simulink model "HANcoder_E407_TTA_Controller_v4_7"  (R2018b)
settings: Solver=FixedStepDiscrete  StartTime=0.0  StopTime=1  FixedStep=0.01  RelTol=1e-3
PreLoadFcn:
  | librarySetup
  | eval([bdroot,'_startup']) %Calling [modelName]_startup.m
values from neighbouring files (symbols this model uses):
  Backup_Board = 0    [HANcoder_E407_TTA_Controller_v3_5_startup.m]    (also in HANcoder_E407_TTA_Controller_v4_6_startup.m; HANcoder_E407_TTA_Controller_v4_7_startup.m; HANcoder_E407_TTA_Controller_v4_startup.m)
  basic_cycle_duration_bc0 = TM_Reset_Board   + COMP_duration    (= 212)    [HANcoder_E407_TTA_Controller_v3_5_startup.m]    (also in HANcoder_E407_TTA_Controller_v4_6_startup.m; HANcoder_E407_TTA_Controller_v4_7_startup.m; HANcoder_E407_TTA_Controller_v4_startup.m)
  basic_cycle_duration_bc1 = TM_Reset_Var_bc1 + COMP_duration    (= 288)    [HANcoder_E407_TTA_Controller_v3_5_startup.m]    (also in HANcoder_E407_TTA_Controller_v4_6_startup.m = 332; HANcoder_E407_TTA_Controller_v4_7_startup.m = 372; HANcoder_E407_TTA_Controller_v4_startup.m = 332)
  comm_delay_estimation1 = round(comm_delay_measured1*hardware_granularity/frequency_IRQ)    [HANcoder_E407_TTA_Controller_v3_5_startup.m]    (also in HANcoder_E407_TTA_Controller_v4_6_startup.m; HANcoder_E407_TTA_Controller_v4_7_startup.m; HANcoder_E407_TTA_Controller_v4_startup.m)
  comm_delay_estimation2 = round(comm_delay_measured2*hardware_granularity/frequency_IRQ)    [HANcoder_E407_TTA_Controller_v3_5_startup.m]    (also in HANcoder_E407_TTA_Controller_v4_6_startup.m; HANcoder_E407_TTA_Controller_v4_7_startup.m; HANcoder_E407_TTA_Controller_v4_startup.m)
  COMM_Period = 40    [HANcoder_E407_TTA_Controller_v3_5_startup.m]    (also in HANcoder_E407_TTA_Controller_v4_6_startup.m; HANcoder_E407_TTA_Controller_v4_7_startup.m; HANcoder_E407_TTA_Controller_v4_startup.m)
  COMM_Phase1 = Simulink.Parameter    [HANcoder_E407_TTA_Controller_v3_5_startup.m]    (also in HANcoder_E407_TTA_Controller_v4_6_startup.m; HANcoder_E407_TTA_Controller_v4_7_startup.m; HANcoder_E407_TTA_Controller_v4_startup.m)
  COMM_Phase2 = Simulink.Parameter    [HANcoder_E407_TTA_Controller_v3_5_startup.m]    (also in HANcoder_E407_TTA_Controller_v4_6_startup.m; HANcoder_E407_TTA_Controller_v4_7_startup.m; HANcoder_E407_TTA_Controller_v4_startup.m)
  COMM_Phase_init1 = Simulink.Parameter    [HANcoder_E407_TTA_Controller_v3_5_startup.m]    (also in HANcoder_E407_TTA_Controller_v4_6_startup.m; HANcoder_E407_TTA_Controller_v4_7_startup.m; HANcoder_E407_TTA_Controller_v4_startup.m)
  COMM_Phase_init2 = Simulink.Parameter    [HANcoder_E407_TTA_Controller_v3_5_startup.m]    (also in HANcoder_E407_TTA_Controller_v4_6_startup.m; HANcoder_E407_TTA_Controller_v4_7_startup.m; HANcoder_E407_TTA_Controller_v4_startup.m)
  COMP_duration = 4    [HANcoder_E407_TTA_Controller_v3_5_startup.m]    (also in HANcoder_E407_TTA_Controller_v4_6_startup.m; HANcoder_E407_TTA_Controller_v4_7_startup.m; HANcoder_E407_TTA_Controller_v4_startup.m)
  Controller1_Board = 1    [HANcoder_E407_TTA_Controller_v3_5_startup.m]    (also in HANcoder_E407_TTA_Controller_v4_6_startup.m; HANcoder_E407_TTA_Controller_v4_7_startup.m; HANcoder_E407_TTA_Controller_v4_startup.m)
  Controller2_Board = 2    [HANcoder_E407_TTA_Controller_v3_5_startup.m]    (also in HANcoder_E407_TTA_Controller_v4_6_startup.m; HANcoder_E407_TTA_Controller_v4_7_startup.m; HANcoder_E407_TTA_Controller_v4_startup.m)
  Controller3_Board = 3    [HANcoder_E407_TTA_Controller_v3_5_startup.m]    (also in HANcoder_E407_TTA_Controller_v4_6_startup.m; HANcoder_E407_TTA_Controller_v4_7_startup.m; HANcoder_E407_TTA_Controller_v4_startup.m)
  delta_a_set = Simulink.Parameter    [HANcoder_E407_TTA_Controller_v3_5_startup.m]    (also in HANcoder_E407_TTA_Controller_v4_6_startup.m; HANcoder_E407_TTA_Controller_v4_7_startup.m; HANcoder_E407_TTA_Controller_v4_startup.m)
  delta_f_set = Simulink.Parameter    [HANcoder_E407_TTA_Controller_v3_5_startup.m]    (also in HANcoder_E407_TTA_Controller_v4_6_startup.m; HANcoder_E407_TTA_Controller_v4_7_startup.m; HANcoder_E407_TTA_Controller_v4_startup.m)
  delta_max = 1    [HANcoder_E407_TTA_Controller_v3_5_startup.m]    (also in HANcoder_E407_TTA_Controller_v4_6_startup.m; HANcoder_E407_TTA_Controller_v4_7_startup.m; HANcoder_E407_TTA_Controller_v4_startup.m)
  delta_min = -1    [HANcoder_E407_TTA_Controller_v3_5_startup.m]    (also in HANcoder_E407_TTA_Controller_v4_6_startup.m; HANcoder_E407_TTA_Controller_v4_7_startup.m; HANcoder_E407_TTA_Controller_v4_startup.m)
  delta_precision = 6    [HANcoder_E407_TTA_Controller_v3_5_startup.m]    (also in HANcoder_E407_TTA_Controller_v4_6_startup.m; HANcoder_E407_TTA_Controller_v4_7_startup.m; HANcoder_E407_TTA_Controller_v4_startup.m)
  e_width = 0.1    [HANcoder_E407_TTA_Controller_v3_5_startup.m]    (also in HANcoder_E407_TTA_Controller_v4_6_startup.m; HANcoder_E407_TTA_Controller_v4_7_startup.m; HANcoder_E407_TTA_Controller_v4_startup.m)
  frequency_IRQ = 100    [HANcoder_E407_2xCAN_TEST_startup.m]    (also in HANcoder_E407_TTA_Controller_v3_5_startup.m; HANcoder_E407_TTA_Controller_v4_6_startup.m; HANcoder_E407_TTA_Controller_v4_7_startup.m; HANcoder_E407_TTA_Controller_v4_startup.m)
  HANtuneOverride = Simulink.Parameter    [HANcoder_E407_2xCAN_TEST_startup.m]    (also in HANcoder_E407_TTA_Controller_v3_5_startup.m; HANcoder_E407_TTA_Controller_v4_6_startup.m; HANcoder_E407_TTA_Controller_v4_7_startup.m; HANcoder_E407_TTA_Controller_v4_startup.m)
  hardware_granularity = 1000000    [HANcoder_E407_2xCAN_TEST_startup.m]    (also in HANcoder_E407_TTA_Controller_v3_5_startup.m; HANcoder_E407_TTA_Controller_v4_6_startup.m; HANcoder_E407_TTA_Controller_v4_7_startup.m; HANcoder_E407_TTA_Controller_v4_startup.m)
  I_a = 2.25    [HANcoder_E407_TTA_Controller_v3_5_startup.m]    (also in HANcoder_E407_TTA_Controller_v4_6_startup.m; HANcoder_E407_TTA_Controller_v4_7_startup.m; HANcoder_E407_TTA_Controller_v4_startup.m)
  I_f = 2.25    [HANcoder_E407_TTA_Controller_v3_5_startup.m]    (also in HANcoder_E407_TTA_Controller_v4_6_startup.m; HANcoder_E407_TTA_Controller_v4_7_startup.m; HANcoder_E407_TTA_Controller_v4_startup.m)
  idle_time_init = basic_cycle_duration_bc0 + basic_cycle_duration_bc1    (= 500)    [HANcoder_E407_TTA_Controller_v3_5_startup.m]    (also in HANcoder_E407_TTA_Controller_v4_6_startup.m = 544; HANcoder_E407_TTA_Controller_v4_7_startup.m = 584; HANcoder_E407_TTA_Controller_v4_startup.m = 544)
  Input_Gen_Board = 4    [HANcoder_E407_TTA_Controller_v3_5_startup.m]    (also in HANcoder_E407_TTA_Controller_v4_6_startup.m; HANcoder_E407_TTA_Controller_v4_7_startup.m; HANcoder_E407_TTA_Controller_v4_startup.m)
  LA_Clock_Gr = 1    [HANcoder_E407_TTA_Controller_v3_5_startup.m]    (also in HANcoder_E407_TTA_Controller_v4_6_startup.m; HANcoder_E407_TTA_Controller_v4_7_startup.m; HANcoder_E407_TTA_Controller_v4_startup.m)
  LA_COMM_dly = 1    [HANcoder_E407_TTA_Controller_v3_5_startup.m]    (also in HANcoder_E407_TTA_Controller_v4_6_startup.m; HANcoder_E407_TTA_Controller_v4_7_startup.m; HANcoder_E407_TTA_Controller_v4_startup.m)
  LA_COMM_Err = 1    [HANcoder_E407_TTA_Controller_v3_5_startup.m]    (also in HANcoder_E407_TTA_Controller_v4_6_startup.m; HANcoder_E407_TTA_Controller_v4_7_startup.m; HANcoder_E407_TTA_Controller_v4_startup.m)
  LA_E_Desync = 1    [HANcoder_E407_TTA_Controller_v3_5_startup.m]    (also in HANcoder_E407_TTA_Controller_v4_6_startup.m; HANcoder_E407_TTA_Controller_v4_7_startup.m; HANcoder_E407_TTA_Controller_v4_startup.m)
  LA_MEX_Flag = 1    [HANcoder_E407_TTA_Controller_v3_5_startup.m]    (also in HANcoder_E407_TTA_Controller_v4_6_startup.m; HANcoder_E407_TTA_Controller_v4_7_startup.m; HANcoder_E407_TTA_Controller_v4_startup.m)
  LA_Task_Act = 1    [HANcoder_E407_TTA_Controller_v3_5_startup.m]    (also in HANcoder_E407_TTA_Controller_v4_6_startup.m; HANcoder_E407_TTA_Controller_v4_7_startup.m; HANcoder_E407_TTA_Controller_v4_startup.m)
  m_v = 100.0    (= 100)    [HANcoder_E407_TTA_Controller_v3_5_startup.m]    (also in HANcoder_E407_TTA_Controller_v4_6_startup.m; HANcoder_E407_TTA_Controller_v4_7_startup.m; HANcoder_E407_TTA_Controller_v4_startup.m)
  Master_Role = 1    [HANcoder_E407_TTA_Controller_v3_5_startup.m]    (also in HANcoder_E407_TTA_Controller_v4_6_startup.m; HANcoder_E407_TTA_Controller_v4_7_startup.m; HANcoder_E407_TTA_Controller_v4_startup.m)
  matrix_cycle_duration = basic_cycle_duration_bc0 + basic_cycle_duration_bc1    (= 500)    [HANcoder_E407_TTA_Controller_v3_5_startup.m]    (also in HANcoder_E407_TTA_Controller_v4_6_startup.m = 544; HANcoder_E407_TTA_Controller_v4_7_startup.m = 584; HANcoder_E407_TTA_Controller_v4_startup.m = 544)
  matrix_rows = 2    [HANcoder_E407_TTA_Controller_v3_5_startup.m]    (also in HANcoder_E407_TTA_Controller_v4_6_startup.m; HANcoder_E407_TTA_Controller_v4_7_startup.m; HANcoder_E407_TTA_Controller_v4_startup.m)
  max_desync = 15    [HANcoder_E407_TTA_Controller_v3_5_startup.m]    (also in HANcoder_E407_TTA_Controller_v4_6_startup.m; HANcoder_E407_TTA_Controller_v4_7_startup.m = 30; HANcoder_E407_TTA_Controller_v4_startup.m)
  max_num_msgs_CAN1 = 2^Tx_bit_number-1    (= 7)    [HANcoder_E407_TTA_Controller_v3_5_startup.m]    (also in HANcoder_E407_TTA_Controller_v4_6_startup.m = 15; HANcoder_E407_TTA_Controller_v4_7_startup.m = 15; HANcoder_E407_TTA_Controller_v4_startup.m)
  max_num_msgs_CAN2 = max_num_msgs_CAN1    (= 7)    [HANcoder_E407_TTA_Controller_v3_5_startup.m]    (also in HANcoder_E407_TTA_Controller_v4_6_startup.m = 15; HANcoder_E407_TTA_Controller_v4_7_startup.m = 15; HANcoder_E407_TTA_Controller_v4_startup.m)
  min_desync = (-1)*max_desync    (= -15)    [HANcoder_E407_TTA_Controller_v3_5_startup.m]    (also in HANcoder_E407_TTA_Controller_v4_6_startup.m; HANcoder_E407_TTA_Controller_v4_7_startup.m = -30; HANcoder_E407_TTA_Controller_v4_startup.m)
  OutControl1_ID = 23    [HANcoder_E407_TTA_Controller_v3_5_startup.m]    (also in HANcoder_E407_TTA_Controller_v4_6_startup.m; HANcoder_E407_TTA_Controller_v4_7_startup.m; HANcoder_E407_TTA_Controller_v4_startup.m)
  OutControl2_ID = 24    [HANcoder_E407_TTA_Controller_v3_5_startup.m]    (also in HANcoder_E407_TTA_Controller_v4_6_startup.m; HANcoder_E407_TTA_Controller_v4_7_startup.m; HANcoder_E407_TTA_Controller_v4_startup.m)
  OutEmulator_ID = 25    [HANcoder_E407_TTA_Controller_v3_5_startup.m]    (also in HANcoder_E407_TTA_Controller_v4_6_startup.m = 26; HANcoder_E407_TTA_Controller_v4_7_startup.m = 26; HANcoder_E407_TTA_Controller_v4_startup.m)
  OutMaster_ID = 25    [HANcoder_E407_TTA_Controller_v4_6_startup.m]    (also in HANcoder_E407_TTA_Controller_v4_7_startup.m; HANcoder_E407_TTA_Controller_v4_startup.m = 26)
  R_al = 0.10    (= 0.1)    [HANcoder_E407_TTA_Controller_v3_5_startup.m]    (also in HANcoder_E407_TTA_Controller_v4_6_startup.m; HANcoder_E407_TTA_Controller_v4_7_startup.m; HANcoder_E407_TTA_Controller_v4_startup.m)
  R_ar = 0.10    (= 0.1)    [HANcoder_E407_TTA_Controller_v3_5_startup.m]    (also in HANcoder_E407_TTA_Controller_v4_6_startup.m; HANcoder_E407_TTA_Controller_v4_7_startup.m; HANcoder_E407_TTA_Controller_v4_startup.m)
  R_fl = 0.10    (= 0.1)    [HANcoder_E407_TTA_Controller_v3_5_startup.m]    (also in HANcoder_E407_TTA_Controller_v4_6_startup.m; HANcoder_E407_TTA_Controller_v4_7_startup.m; HANcoder_E407_TTA_Controller_v4_startup.m)
  R_fr = 0.10    (= 0.1)    [HANcoder_E407_TTA_Controller_v3_5_startup.m]    (also in HANcoder_E407_TTA_Controller_v4_6_startup.m; HANcoder_E407_TTA_Controller_v4_7_startup.m; HANcoder_E407_TTA_Controller_v4_startup.m)
  script_run = Simulink.Parameter    [HANcoder_E407_TTA_Controller_v3_5_startup.m]    (also in HANcoder_E407_TTA_Controller_v4_6_startup.m; HANcoder_E407_TTA_Controller_v4_7_startup.m; HANcoder_E407_TTA_Controller_v4_startup.m)
  SensorValues_ID = 22    [HANcoder_E407_TTA_Controller_v3_5_startup.m]    (also in HANcoder_E407_TTA_Controller_v4_6_startup.m; HANcoder_E407_TTA_Controller_v4_7_startup.m; HANcoder_E407_TTA_Controller_v4_startup.m)
  SetValues_ID = 21    [HANcoder_E407_TTA_Controller_v3_5_startup.m]    (also in HANcoder_E407_TTA_Controller_v4_6_startup.m; HANcoder_E407_TTA_Controller_v4_7_startup.m; HANcoder_E407_TTA_Controller_v4_startup.m)
  Slave_Role = 2    [HANcoder_E407_TTA_Controller_v3_5_startup.m]    (also in HANcoder_E407_TTA_Controller_v4_6_startup.m; HANcoder_E407_TTA_Controller_v4_7_startup.m; HANcoder_E407_TTA_Controller_v4_startup.m)
  speed_k_d = Simulink.Parameter    [HANcoder_E407_TTA_Controller_v3_5_startup.m]    (also in HANcoder_E407_TTA_Controller_v4_6_startup.m; HANcoder_E407_TTA_Controller_v4_7_startup.m; HANcoder_E407_TTA_Controller_v4_startup.m)
  speed_k_i = Simulink.Parameter    [HANcoder_E407_TTA_Controller_v3_5_startup.m]    (also in HANcoder_E407_TTA_Controller_v4_6_startup.m; HANcoder_E407_TTA_Controller_v4_7_startup.m; HANcoder_E407_TTA_Controller_v4_startup.m)
  speed_k_p = Simulink.Parameter    [HANcoder_E407_TTA_Controller_v3_5_startup.m]    (also in HANcoder_E407_TTA_Controller_v4_6_startup.m; HANcoder_E407_TTA_Controller_v4_7_startup.m; HANcoder_E407_TTA_Controller_v4_startup.m)
  speed_max = 10    [HANcoder_E407_TTA_Controller_v3_5_startup.m]    (also in HANcoder_E407_TTA_Controller_v4_6_startup.m; HANcoder_E407_TTA_Controller_v4_7_startup.m; HANcoder_E407_TTA_Controller_v4_startup.m)
  speed_min = -10    [HANcoder_E407_TTA_Controller_v3_5_startup.m]    (also in HANcoder_E407_TTA_Controller_v4_6_startup.m; HANcoder_E407_TTA_Controller_v4_7_startup.m; HANcoder_E407_TTA_Controller_v4_startup.m)
  speed_precision = 3    [HANcoder_E407_TTA_Controller_v3_5_startup.m]    (also in HANcoder_E407_TTA_Controller_v4_6_startup.m; HANcoder_E407_TTA_Controller_v4_7_startup.m; HANcoder_E407_TTA_Controller_v4_startup.m)
  Sync_ID = 1    [HANcoder_E407_TTA_Controller_v3_5_startup.m]    (also in HANcoder_E407_TTA_Controller_v4_6_startup.m; HANcoder_E407_TTA_Controller_v4_7_startup.m; HANcoder_E407_TTA_Controller_v4_startup.m)
  tau_max = 5    [HANcoder_E407_TTA_Controller_v3_5_startup.m]    (also in HANcoder_E407_TTA_Controller_v4_6_startup.m; HANcoder_E407_TTA_Controller_v4_7_startup.m; HANcoder_E407_TTA_Controller_v4_startup.m)
  tau_min = -5    [HANcoder_E407_TTA_Controller_v3_5_startup.m]    (also in HANcoder_E407_TTA_Controller_v4_6_startup.m; HANcoder_E407_TTA_Controller_v4_7_startup.m; HANcoder_E407_TTA_Controller_v4_startup.m)
  tau_range = abs(tau_max) + abs(tau_min)    [HANcoder_E407_TTA_Controller_v3_5_startup.m]    (also in HANcoder_E407_TTA_Controller_v4_6_startup.m; HANcoder_E407_TTA_Controller_v4_7_startup.m; HANcoder_E407_TTA_Controller_v4_startup.m)
  theta_max = (speed_max/R_fr)*matrix_cycle_duration*frequency_IRQ/hardware_granularity    (= 5)    [HANcoder_E407_TTA_Controller_v3_5_startup.m]    (also in HANcoder_E407_TTA_Controller_v4_6_startup.m = 5.44; HANcoder_E407_TTA_Controller_v4_7_startup.m = 5.84; HANcoder_E407_TTA_Controller_v4_startup.m = 5.44)
  theta_min = (-1)*theta_max    (= -5)    [HANcoder_E407_TTA_Controller_v3_5_startup.m]    (also in HANcoder_E407_TTA_Controller_v4_6_startup.m = -5.44; HANcoder_E407_TTA_Controller_v4_7_startup.m = -5.84; HANcoder_E407_TTA_Controller_v4_startup.m = -5.44)
  theta_precision = 7-(fix(log2(theta_max))+1)    [HANcoder_E407_TTA_Controller_v3_5_startup.m]    (also in HANcoder_E407_TTA_Controller_v4_6_startup.m; HANcoder_E407_TTA_Controller_v4_7_startup.m; HANcoder_E407_TTA_Controller_v4_startup.m)
  Tl_a = 0.6    [HANcoder_E407_TTA_Controller_v3_5_startup.m]    (also in HANcoder_E407_TTA_Controller_v4_6_startup.m; HANcoder_E407_TTA_Controller_v4_7_startup.m; HANcoder_E407_TTA_Controller_v4_startup.m)
  Tl_f = 0.6    [HANcoder_E407_TTA_Controller_v3_5_startup.m]    (also in HANcoder_E407_TTA_Controller_v4_6_startup.m; HANcoder_E407_TTA_Controller_v4_7_startup.m; HANcoder_E407_TTA_Controller_v4_startup.m)
  TM_Check_Output_Control1 = TM_COMM_Output_Control1 + COMM_duration    (= 188)    [HANcoder_E407_TTA_Controller_v3_5_startup.m]    (also in HANcoder_E407_TTA_Controller_v4_6_startup.m; HANcoder_E407_TTA_Controller_v4_7_startup.m; HANcoder_E407_TTA_Controller_v4_startup.m)
  TM_Check_Output_Control2 = TM_COMM_Output_Control2 + COMM_duration    (= 232)    [HANcoder_E407_TTA_Controller_v3_5_startup.m]    (also in HANcoder_E407_TTA_Controller_v4_6_startup.m; HANcoder_E407_TTA_Controller_v4_7_startup.m; HANcoder_E407_TTA_Controller_v4_startup.m)
  TM_Check_Output_Emulator = TM_COMM_Output_Emulator + COMM_duration    (= 280)    [HANcoder_E407_TTA_Controller_v3_5_startup.m]    (also in HANcoder_E407_TTA_Controller_v4_6_startup.m = 320; HANcoder_E407_TTA_Controller_v4_7_startup.m = 360; HANcoder_E407_TTA_Controller_v4_startup.m = 320)
  TM_Check_Output_Emulator_2 = TM_Check_Output_Emulator + 2    (= 282)    [HANcoder_E407_TTA_Controller_v3_5_startup.m]    (also in HANcoder_E407_TTA_Controller_v4_6_startup.m = 322; HANcoder_E407_TTA_Controller_v4_7_startup.m = 362; HANcoder_E407_TTA_Controller_v4_startup.m = 322)
  TM_Check_Output_Emulator_3 = TM_Check_Output_Emulator_2 + 2    (= 324)    [HANcoder_E407_TTA_Controller_v4_6_startup.m]    (also in HANcoder_E407_TTA_Controller_v4_7_startup.m = 364; HANcoder_E407_TTA_Controller_v4_startup.m)
  TM_Check_Output_Master = TM_COMM_Output_Master + COMM_duration    (= 312)    [HANcoder_E407_TTA_Controller_v4_7_startup.m]
  TM_Check_Sensor_Values = TM_COMM_Sensor_Values + COMM_duration    (= 132)    [HANcoder_E407_TTA_Controller_v3_5_startup.m]    (also in HANcoder_E407_TTA_Controller_v4_6_startup.m; HANcoder_E407_TTA_Controller_v4_7_startup.m; HANcoder_E407_TTA_Controller_v4_startup.m)
  TM_Check_Sensor_Values_2 = TM_Check_Sensor_Values + 2    (= 134)    [HANcoder_E407_TTA_Controller_v3_5_startup.m]    (also in HANcoder_E407_TTA_Controller_v4_6_startup.m; HANcoder_E407_TTA_Controller_v4_7_startup.m; HANcoder_E407_TTA_Controller_v4_startup.m)
  TM_Check_Set_Values = TM_COMM_Set_Values + COMM_duration    (= 88)    [HANcoder_E407_TTA_Controller_v3_5_startup.m]    (also in HANcoder_E407_TTA_Controller_v4_6_startup.m; HANcoder_E407_TTA_Controller_v4_7_startup.m; HANcoder_E407_TTA_Controller_v4_startup.m)
  TM_Check_Set_Values_2 = TM_Check_Set_Values + 2    (= 90)    [HANcoder_E407_TTA_Controller_v3_5_startup.m]    (also in HANcoder_E407_TTA_Controller_v4_6_startup.m; HANcoder_E407_TTA_Controller_v4_7_startup.m; HANcoder_E407_TTA_Controller_v4_startup.m)
  TM_Check_Sync = TM_COMM_Sync   + COMM_duration    (= 40)    [HANcoder_E407_TTA_Controller_v3_5_startup.m]    (also in HANcoder_E407_TTA_Controller_v4_6_startup.m; HANcoder_E407_TTA_Controller_v4_7_startup.m; HANcoder_E407_TTA_Controller_v4_startup.m)
  TM_Check_TOuts = TM_Count_Vote3 + COMP_duration    (= 196)    [HANcoder_E407_TTA_Controller_v3_5_startup.m]    (also in HANcoder_E407_TTA_Controller_v4_6_startup.m; HANcoder_E407_TTA_Controller_v4_7_startup.m; HANcoder_E407_TTA_Controller_v4_startup.m)
  TM_Check_Vote1 = TM_COMM_Vote1  + COMM_duration    (= 92)    [HANcoder_E407_TTA_Controller_v3_5_startup.m]    (also in HANcoder_E407_TTA_Controller_v4_6_startup.m; HANcoder_E407_TTA_Controller_v4_7_startup.m; HANcoder_E407_TTA_Controller_v4_startup.m)
  TM_Check_Vote2 = TM_COMM_Vote2  + COMM_duration    (= 140)    [HANcoder_E407_TTA_Controller_v3_5_startup.m]    (also in HANcoder_E407_TTA_Controller_v4_6_startup.m; HANcoder_E407_TTA_Controller_v4_7_startup.m; HANcoder_E407_TTA_Controller_v4_startup.m)
  TM_Check_Vote2_2 = TM_Check_Vote2 + 2    (= 142)    [HANcoder_E407_TTA_Controller_v3_5_startup.m]    (also in HANcoder_E407_TTA_Controller_v4_6_startup.m; HANcoder_E407_TTA_Controller_v4_7_startup.m; HANcoder_E407_TTA_Controller_v4_startup.m)
  TM_Check_Vote3 = TM_COMM_Vote3  + COMM_duration    (= 188)    [HANcoder_E407_TTA_Controller_v3_5_startup.m]    (also in HANcoder_E407_TTA_Controller_v4_6_startup.m; HANcoder_E407_TTA_Controller_v4_7_startup.m; HANcoder_E407_TTA_Controller_v4_startup.m)
  TM_COMM_Output_Control1 = TM_Velocity + COMP_duration    (= 148)    [HANcoder_E407_TTA_Controller_v3_5_startup.m]    (also in HANcoder_E407_TTA_Controller_v4_6_startup.m; HANcoder_E407_TTA_Controller_v4_7_startup.m; HANcoder_E407_TTA_Controller_v4_startup.m)
  TM_COMM_Output_Control2 = TM_Check_Output_Control1 + COMP_duration    (= 192)    [HANcoder_E407_TTA_Controller_v3_5_startup.m]    (also in HANcoder_E407_TTA_Controller_v4_6_startup.m; HANcoder_E407_TTA_Controller_v4_7_startup.m; HANcoder_E407_TTA_Controller_v4_startup.m)
  TM_COMM_Output_Emulator = TM_TMR + COMP_duration    (= 240)    [HANcoder_E407_TTA_Controller_v3_5_startup.m]    (also in HANcoder_E407_TTA_Controller_v4_6_startup.m = 280; HANcoder_E407_TTA_Controller_v4_7_startup.m = 320; HANcoder_E407_TTA_Controller_v4_startup.m = 280)
  TM_COMM_Output_Master = TM_Check_Output_Control2 + COMM_duration    (= 272)    [HANcoder_E407_TTA_Controller_v4_6_startup.m]    (also in HANcoder_E407_TTA_Controller_v4_7_startup.m; HANcoder_E407_TTA_Controller_v4_startup.m)
  TM_COMM_Sensor_Values = TM_Check_Set_Values + COMP_duration    (= 92)    [HANcoder_E407_TTA_Controller_v3_5_startup.m]    (also in HANcoder_E407_TTA_Controller_v4_6_startup.m; HANcoder_E407_TTA_Controller_v4_7_startup.m; HANcoder_E407_TTA_Controller_v4_startup.m)
  TM_COMM_Set_Values = TM_Update_LT + COMP_duration    (= 48)    [HANcoder_E407_TTA_Controller_v3_5_startup.m]    (also in HANcoder_E407_TTA_Controller_v4_6_startup.m; HANcoder_E407_TTA_Controller_v4_7_startup.m; HANcoder_E407_TTA_Controller_v4_startup.m)
  TM_COMM_Sync = basic_cycle_start    (= 0)    [HANcoder_E407_TTA_Controller_v3_5_startup.m]    (also in HANcoder_E407_TTA_Controller_v4_6_startup.m; HANcoder_E407_TTA_Controller_v4_7_startup.m; HANcoder_E407_TTA_Controller_v4_startup.m)
  TM_COMM_Vote1 = TM_Vote_Dec    + COMP_duration    (= 52)    [HANcoder_E407_TTA_Controller_v3_5_startup.m]    (also in HANcoder_E407_TTA_Controller_v4_6_startup.m; HANcoder_E407_TTA_Controller_v4_7_startup.m; HANcoder_E407_TTA_Controller_v4_startup.m)
  TM_COMM_Vote2 = TM_Count_Vote1 + COMP_duration    (= 100)    [HANcoder_E407_TTA_Controller_v3_5_startup.m]    (also in HANcoder_E407_TTA_Controller_v4_6_startup.m; HANcoder_E407_TTA_Controller_v4_7_startup.m; HANcoder_E407_TTA_Controller_v4_startup.m)
  TM_COMM_Vote3 = TM_Count_Vote2 + COMP_duration    (= 148)    [HANcoder_E407_TTA_Controller_v3_5_startup.m]    (also in HANcoder_E407_TTA_Controller_v4_6_startup.m; HANcoder_E407_TTA_Controller_v4_7_startup.m; HANcoder_E407_TTA_Controller_v4_startup.m)
  TM_Count_Vote1 = TM_Check_Vote1 + COMP_duration    (= 96)    [HANcoder_E407_TTA_Controller_v3_5_startup.m]    (also in HANcoder_E407_TTA_Controller_v4_6_startup.m; HANcoder_E407_TTA_Controller_v4_7_startup.m; HANcoder_E407_TTA_Controller_v4_startup.m)
  TM_Count_Vote2 = TM_Check_Vote2 + COMP_duration    (= 144)    [HANcoder_E407_TTA_Controller_v3_5_startup.m]    (also in HANcoder_E407_TTA_Controller_v4_6_startup.m; HANcoder_E407_TTA_Controller_v4_7_startup.m; HANcoder_E407_TTA_Controller_v4_startup.m)
  TM_Count_Vote3 = TM_Check_Vote3 + COMP_duration    (= 192)    [HANcoder_E407_TTA_Controller_v3_5_startup.m]    (also in HANcoder_E407_TTA_Controller_v4_6_startup.m; HANcoder_E407_TTA_Controller_v4_7_startup.m; HANcoder_E407_TTA_Controller_v4_startup.m)
  TM_Data_bc0 = TM_COMM_Sync    (= 0)    [HANcoder_E407_TTA_Controller_v3_5_startup.m]    (also in HANcoder_E407_TTA_Controller_v4_6_startup.m; HANcoder_E407_TTA_Controller_v4_7_startup.m; HANcoder_E407_TTA_Controller_v4_startup.m)
  TM_Data_bc1 = TM_Data_bc0(1:4)    [HANcoder_E407_TTA_Controller_v3_5_startup.m]    (also in HANcoder_E407_TTA_Controller_v4_6_startup.m; HANcoder_E407_TTA_Controller_v4_7_startup.m; HANcoder_E407_TTA_Controller_v4_startup.m)
  TM_New_Master = TM_Check_TOuts + COMP_duration    (= 200)    [HANcoder_E407_TTA_Controller_v3_5_startup.m]    (also in HANcoder_E407_TTA_Controller_v4_6_startup.m; HANcoder_E407_TTA_Controller_v4_7_startup.m; HANcoder_E407_TTA_Controller_v4_startup.m)
  TM_Reset_Board = TM_Reset_Var   + COMP_duration    (= 208)    [HANcoder_E407_TTA_Controller_v3_5_startup.m]    (also in HANcoder_E407_TTA_Controller_v4_6_startup.m; HANcoder_E407_TTA_Controller_v4_7_startup.m; HANcoder_E407_TTA_Controller_v4_startup.m)
  TM_Reset_Var = TM_New_Master  + COMP_duration    (= 204)    [HANcoder_E407_TTA_Controller_v3_5_startup.m]    (also in HANcoder_E407_TTA_Controller_v4_6_startup.m; HANcoder_E407_TTA_Controller_v4_7_startup.m; HANcoder_E407_TTA_Controller_v4_startup.m)
  TM_Reset_Var_bc1 = TM_Check_Output_Emulator + COMP_duration    (= 284)    [HANcoder_E407_TTA_Controller_v3_5_startup.m]    (also in HANcoder_E407_TTA_Controller_v4_6_startup.m = 328; HANcoder_E407_TTA_Controller_v4_7_startup.m = 368; HANcoder_E407_TTA_Controller_v4_startup.m = 328)
  TM_Reset_Var_bc1_2 = TM_Reset_Var_bc1 + 2    (= 286)    [HANcoder_E407_TTA_Controller_v3_5_startup.m]    (also in HANcoder_E407_TTA_Controller_v4_6_startup.m = 330; HANcoder_E407_TTA_Controller_v4_7_startup.m = 370; HANcoder_E407_TTA_Controller_v4_startup.m = 330)
  TM_Steer = TM_Check_Sensor_Values + COMP_duration    (= 136)    [HANcoder_E407_TTA_Controller_v3_5_startup.m]    (also in HANcoder_E407_TTA_Controller_v4_6_startup.m; HANcoder_E407_TTA_Controller_v4_7_startup.m; HANcoder_E407_TTA_Controller_v4_startup.m)
  TM_TMR = TM_Check_Output_Control2 + COMP_duration    (= 236)    [HANcoder_E407_TTA_Controller_v3_5_startup.m]    (also in HANcoder_E407_TTA_Controller_v4_6_startup.m = 276; HANcoder_E407_TTA_Controller_v4_7_startup.m = 316; HANcoder_E407_TTA_Controller_v4_startup.m = 276)
  TM_TMR_2 = TM_TMR + 1    (= 237)    [HANcoder_E407_TTA_Controller_v3_5_startup.m]    (also in HANcoder_E407_TTA_Controller_v4_6_startup.m = 277; HANcoder_E407_TTA_Controller_v4_7_startup.m = 317; HANcoder_E407_TTA_Controller_v4_startup.m = 277)
  TM_TMR_3 = TM_TMR + 3    (= 239)    [HANcoder_E407_TTA_Controller_v3_5_startup.m]    (also in HANcoder_E407_TTA_Controller_v4_6_startup.m = 279; HANcoder_E407_TTA_Controller_v4_7_startup.m = 319; HANcoder_E407_TTA_Controller_v4_startup.m = 279)
  TM_Torque = TM_Steer + COMP_duration    (= 140)    [HANcoder_E407_TTA_Controller_v3_5_startup.m]    (also in HANcoder_E407_TTA_Controller_v4_6_startup.m; HANcoder_E407_TTA_Controller_v4_7_startup.m; HANcoder_E407_TTA_Controller_v4_startup.m)
  TM_Type_bc0 = COMM    (= 0)    [HANcoder_E407_TTA_Controller_v3_5_startup.m]    (also in HANcoder_E407_TTA_Controller_v4_6_startup.m; HANcoder_E407_TTA_Controller_v4_7_startup.m; HANcoder_E407_TTA_Controller_v4_startup.m)
  TM_Type_bc1 = TM_Type_bc0(1:4)    [HANcoder_E407_TTA_Controller_v3_5_startup.m]    (also in HANcoder_E407_TTA_Controller_v4_6_startup.m; HANcoder_E407_TTA_Controller_v4_7_startup.m; HANcoder_E407_TTA_Controller_v4_startup.m)
  TM_Update_LT = TM_Check_Sync  + COMP_duration    (= 44)    [HANcoder_E407_TTA_Controller_v3_5_startup.m]    (also in HANcoder_E407_TTA_Controller_v4_6_startup.m; HANcoder_E407_TTA_Controller_v4_7_startup.m; HANcoder_E407_TTA_Controller_v4_startup.m)
  TM_Update_LT_2 = TM_Update_LT   + 2    (= 46)    [HANcoder_E407_TTA_Controller_v3_5_startup.m]    (also in HANcoder_E407_TTA_Controller_v4_6_startup.m; HANcoder_E407_TTA_Controller_v4_7_startup.m; HANcoder_E407_TTA_Controller_v4_startup.m)
  TM_Velocity = TM_Torque + COMP_duration    (= 144)    [HANcoder_E407_TTA_Controller_v3_5_startup.m]    (also in HANcoder_E407_TTA_Controller_v4_6_startup.m; HANcoder_E407_TTA_Controller_v4_7_startup.m; HANcoder_E407_TTA_Controller_v4_startup.m)
  TM_Vote_Dec = TM_Update_LT   + COMP_duration    (= 48)    [HANcoder_E407_TTA_Controller_v3_5_startup.m]    (also in HANcoder_E407_TTA_Controller_v4_6_startup.m; HANcoder_E407_TTA_Controller_v4_7_startup.m; HANcoder_E407_TTA_Controller_v4_startup.m)
  TM_Vote_Dec_2 = TM_Vote_Dec    + 2    (= 50)    [HANcoder_E407_TTA_Controller_v3_5_startup.m]    (also in HANcoder_E407_TTA_Controller_v4_6_startup.m; HANcoder_E407_TTA_Controller_v4_7_startup.m; HANcoder_E407_TTA_Controller_v4_startup.m)
  torque_a_k_d = Simulink.Parameter    [HANcoder_E407_TTA_Controller_v3_5_startup.m]    (also in HANcoder_E407_TTA_Controller_v4_6_startup.m; HANcoder_E407_TTA_Controller_v4_7_startup.m; HANcoder_E407_TTA_Controller_v4_startup.m)
  torque_a_k_i = Simulink.Parameter    [HANcoder_E407_TTA_Controller_v3_5_startup.m]    (also in HANcoder_E407_TTA_Controller_v4_6_startup.m; HANcoder_E407_TTA_Controller_v4_7_startup.m; HANcoder_E407_TTA_Controller_v4_startup.m)
  torque_a_k_p = Simulink.Parameter    [HANcoder_E407_TTA_Controller_v3_5_startup.m]    (also in HANcoder_E407_TTA_Controller_v4_6_startup.m; HANcoder_E407_TTA_Controller_v4_7_startup.m; HANcoder_E407_TTA_Controller_v4_startup.m)
  torque_f_k_d = Simulink.Parameter    [HANcoder_E407_TTA_Controller_v3_5_startup.m]    (also in HANcoder_E407_TTA_Controller_v4_6_startup.m; HANcoder_E407_TTA_Controller_v4_7_startup.m; HANcoder_E407_TTA_Controller_v4_startup.m)
  ... (+8 more)
undefined symbols (not defined in the file or in its folder): A0, A1, A2, A3, A4, CON2, CON3, CON4, D10, D12, D13, D2, D3, D8, D9
libraries: hdlsllib x477, HANcoder_STM32_Target x30, simulink x3, simulink_extras x1
(part 80 of 80)

== system HANcoder_E407_TTA_Controller_v4_7/HANcoder STM32 Target - E407-STM32 algorithm/TTA CAN System/TTA System/Matrix Cycle Manager/Input Generator Matrix Cycle/input generator basic cycle 1/COMM Task - Set_Values/Transmission subtasks/Check msg transmission CAN1/TX buffer update CAN1/Msg_Data_Encoder ==
  basic_cycle : Inport
  tx_counter : Inport  Port=2
  board_number : Inport  Port=3
  Bit Shift : hdlsllib/Logic and Bit Operations/Bit Shift  mode=Shift Left Logical  N=4
      settings: SourceProductName=HDL Coder  SourceProductBaseCode=HD
  Bit Shift1 : hdlsllib/Logic and Bit Operations/Bit Shift  mode=Shift Left Logical  N=7
      settings: SourceProductName=HDL Coder  SourceProductBaseCode=HD
  Minus : Sum  Inputs=3
  encoded_msg : Outport
  wires:
  basic_cycle/1 -> Bit Shift1/1
  Minus/1 -> encoded_msg/1
  tx_counter/1 -> Bit Shift/1
  Bit Shift1/1 -> Minus/1
  Bit Shift/1 -> Minus/2
  board_number/1 -> Minus/3

== system HANcoder_E407_TTA_Controller_v4_7/HANcoder STM32 Target - E407-STM32 algorithm/TTA CAN System/TTA System/Matrix Cycle Manager/Input Generator Matrix Cycle/input generator basic cycle 1/COMM Task - Set_Values/Transmission subtasks/Check msg transmission CAN2/TX buffer update CAN2/Msg_Data_Encoder ==
  basic_cycle : Inport
  tx_counter : Inport  Port=2
  verif_value : Inport  Port=3
  Bit Shift : hdlsllib/Logic and Bit Operations/Bit Shift  mode=Shift Left Logical  N=4
      settings: SourceProductName=HDL Coder  SourceProductBaseCode=HD
  Bit Shift1 : hdlsllib/Logic and Bit Operations/Bit Shift  mode=Shift Left Logical  N=7
      settings: SourceProductName=HDL Coder  SourceProductBaseCode=HD
  Minus : Sum  Inputs=3
  encoded_msg : Outport
  wires:
  basic_cycle/1 -> Bit Shift1/1
  Minus/1 -> encoded_msg/1
  tx_counter/1 -> Bit Shift/1
  Bit Shift1/1 -> Minus/1
  Bit Shift/1 -> Minus/2
  verif_value/1 -> Minus/3

== system HANcoder_E407_TTA_Controller_v4_7/HANcoder STM32 Target - E407-STM32 algorithm/TTA CAN System/TTA System/Matrix Cycle Manager/Input Generator Matrix Cycle/input generator basic cycle 1/COMM Task - Sync bc 1/Transmission subtasks/Check msg transmission CAN1/TX buffer update CAN1/Msg_Data_Encoder ==
  basic_cycle : Inport
  tx_counter : Inport  Port=2
  board_number : Inport  Port=3
  Bit Shift : hdlsllib/Logic and Bit Operations/Bit Shift  mode=Shift Left Logical  N=4
      settings: SourceProductName=HDL Coder  SourceProductBaseCode=HD
  Bit Shift1 : hdlsllib/Logic and Bit Operations/Bit Shift  mode=Shift Left Logical  N=7
      settings: SourceProductName=HDL Coder  SourceProductBaseCode=HD
  Minus : Sum  Inputs=3
  encoded_msg : Outport
  wires:
  basic_cycle/1 -> Bit Shift1/1
  Minus/1 -> encoded_msg/1
  tx_counter/1 -> Bit Shift/1
  Bit Shift1/1 -> Minus/1
  Bit Shift/1 -> Minus/2
  board_number/1 -> Minus/3

== system HANcoder_E407_TTA_Controller_v4_7/HANcoder STM32 Target - E407-STM32 algorithm/TTA CAN System/TTA System/Matrix Cycle Manager/Input Generator Matrix Cycle/input generator basic cycle 1/COMM Task - Sync bc 1/Transmission subtasks/Check msg transmission CAN2/TX buffer update CAN2/Msg_Data_Encoder ==
  basic_cycle : Inport
  tx_counter : Inport  Port=2
  verif_value : Inport  Port=3
  Bit Shift : hdlsllib/Logic and Bit Operations/Bit Shift  mode=Shift Left Logical  N=4
      settings: SourceProductName=HDL Coder  SourceProductBaseCode=HD
  Bit Shift1 : hdlsllib/Logic and Bit Operations/Bit Shift  mode=Shift Left Logical  N=7
      settings: SourceProductName=HDL Coder  SourceProductBaseCode=HD
  Minus : Sum  Inputs=3
  encoded_msg : Outport
  wires:
  basic_cycle/1 -> Bit Shift1/1
  Minus/1 -> encoded_msg/1
  tx_counter/1 -> Bit Shift/1
  Bit Shift1/1 -> Minus/1
  Bit Shift/1 -> Minus/2
  verif_value/1 -> Minus/3

== system HANcoder_E407_TTA_Controller_v4_7/HANcoder STM32 Target - E407-STM32 algorithm/TTA CAN System/TTA System/Matrix Cycle Manager/Vehicle Emulator Matrix Cycle/vehicle emulator basic cycle 0/COMM Task - Sync bc 0/Transmission subtasks/Check msg transmission CAN1/TX buffer update CAN1/Msg_Data_Encoder ==
  basic_cycle : Inport
  tx_counter : Inport  Port=2
  board_number : Inport  Port=3
  Bit Shift : hdlsllib/Logic and Bit Operations/Bit Shift  mode=Shift Left Logical  N=4
      settings: SourceProductName=HDL Coder  SourceProductBaseCode=HD
  Bit Shift1 : hdlsllib/Logic and Bit Operations/Bit Shift  mode=Shift Left Logical  N=7
      settings: SourceProductName=HDL Coder  SourceProductBaseCode=HD
  Minus : Sum  Inputs=3
  encoded_msg : Outport
  wires:
  basic_cycle/1 -> Bit Shift1/1
  Minus/1 -> encoded_msg/1
  tx_counter/1 -> Bit Shift/1
  Bit Shift1/1 -> Minus/1
  Bit Shift/1 -> Minus/2
  board_number/1 -> Minus/3

== system HANcoder_E407_TTA_Controller_v4_7/HANcoder STM32 Target - E407-STM32 algorithm/TTA CAN System/TTA System/Matrix Cycle Manager/Vehicle Emulator Matrix Cycle/vehicle emulator basic cycle 0/COMM Task - Sync bc 0/Transmission subtasks/Check msg transmission CAN2/TX buffer update CAN2/Msg_Data_Encoder ==
  basic_cycle : Inport
  tx_counter : Inport  Port=2
  verif_value : Inport  Port=3
  Bit Shift : hdlsllib/Logic and Bit Operations/Bit Shift  mode=Shift Left Logical  N=4
      settings: SourceProductName=HDL Coder  SourceProductBaseCode=HD
  Bit Shift1 : hdlsllib/Logic and Bit Operations/Bit Shift  mode=Shift Left Logical  N=7
      settings: SourceProductName=HDL Coder  SourceProductBaseCode=HD
  Minus : Sum  Inputs=3
  encoded_msg : Outport
  wires:
  basic_cycle/1 -> Bit Shift1/1
  Minus/1 -> encoded_msg/1
  tx_counter/1 -> Bit Shift/1
  Bit Shift1/1 -> Minus/1
  Bit Shift/1 -> Minus/2
  verif_value/1 -> Minus/3

== system HANcoder_E407_TTA_Controller_v4_7/HANcoder STM32 Target - E407-STM32 algorithm/TTA CAN System/TTA System/Matrix Cycle Manager/Vehicle Emulator Matrix Cycle/vehicle emulator basic cycle 1/COMM Task - Output Emulator/Transmission subtasks/Check msg transmission CAN1/TX buffer update CAN1/Msg_Data_Encoder ==
  basic_cycle : Inport
  tx_counter : Inport  Port=2
  board_number : Inport  Port=3
  Bit Shift : hdlsllib/Logic and Bit Operations/Bit Shift  mode=Shift Left Logical  N=4
      settings: SourceProductName=HDL Coder  SourceProductBaseCode=HD
  Bit Shift1 : hdlsllib/Logic and Bit Operations/Bit Shift  mode=Shift Left Logical  N=7
      settings: SourceProductName=HDL Coder  SourceProductBaseCode=HD
  Minus : Sum  Inputs=3
  encoded_msg : Outport
  wires:
  basic_cycle/1 -> Bit Shift1/1
  Minus/1 -> encoded_msg/1
  tx_counter/1 -> Bit Shift/1
  Bit Shift1/1 -> Minus/1
  Bit Shift/1 -> Minus/2
  board_number/1 -> Minus/3

== system HANcoder_E407_TTA_Controller_v4_7/HANcoder STM32 Target - E407-STM32 algorithm/TTA CAN System/TTA System/Matrix Cycle Manager/Vehicle Emulator Matrix Cycle/vehicle emulator basic cycle 1/COMM Task - Output Emulator/Transmission subtasks/Check msg transmission CAN2/TX buffer update CAN2/Msg_Data_Encoder ==
  basic_cycle : Inport
  tx_counter : Inport  Port=2
  verif_value : Inport  Port=3
  Bit Shift : hdlsllib/Logic and Bit Operations/Bit Shift  mode=Shift Left Logical  N=4
      settings: SourceProductName=HDL Coder  SourceProductBaseCode=HD
  Bit Shift1 : hdlsllib/Logic and Bit Operations/Bit Shift  mode=Shift Left Logical  N=7
      settings: SourceProductName=HDL Coder  SourceProductBaseCode=HD
  Minus : Sum  Inputs=3
  encoded_msg : Outport
  wires:
  basic_cycle/1 -> Bit Shift1/1
  Minus/1 -> encoded_msg/1
  tx_counter/1 -> Bit Shift/1
  Bit Shift1/1 -> Minus/1
  Bit Shift/1 -> Minus/2
  verif_value/1 -> Minus/3

== system HANcoder_E407_TTA_Controller_v4_7/HANcoder STM32 Target - E407-STM32 algorithm/TTA CAN System/TTA System/Matrix Cycle Manager/Vehicle Emulator Matrix Cycle/vehicle emulator basic cycle 1/COMM Task - Sensor_Values/Transmission subtasks/Check msg transmission CAN1/TX buffer update CAN1/Msg_Data_Encoder ==
  basic_cycle : Inport
  tx_counter : Inport  Port=2
  board_number : Inport  Port=3
  Bit Shift : hdlsllib/Logic and Bit Operations/Bit Shift  mode=Shift Left Logical  N=4
      settings: SourceProductName=HDL Coder  SourceProductBaseCode=HD
  Bit Shift1 : hdlsllib/Logic and Bit Operations/Bit Shift  mode=Shift Left Logical  N=7
      settings: SourceProductName=HDL Coder  SourceProductBaseCode=HD
  Minus : Sum  Inputs=3
  encoded_msg : Outport
  wires:
  basic_cycle/1 -> Bit Shift1/1
  Minus/1 -> encoded_msg/1
  tx_counter/1 -> Bit Shift/1
  Bit Shift1/1 -> Minus/1
  Bit Shift/1 -> Minus/2
  board_number/1 -> Minus/3

== system HANcoder_E407_TTA_Controller_v4_7/HANcoder STM32 Target - E407-STM32 algorithm/TTA CAN System/TTA System/Matrix Cycle Manager/Vehicle Emulator Matrix Cycle/vehicle emulator basic cycle 1/COMM Task - Sensor_Values/Transmission subtasks/Check msg transmission CAN2/TX buffer update CAN2/Msg_Data_Encoder ==
  basic_cycle : Inport
  tx_counter : Inport  Port=2
  verif_value : Inport  Port=3
  Bit Shift : hdlsllib/Logic and Bit Operations/Bit Shift  mode=Shift Left Logical  N=4
      settings: SourceProductName=HDL Coder  SourceProductBaseCode=HD
  Bit Shift1 : hdlsllib/Logic and Bit Operations/Bit Shift  mode=Shift Left Logical  N=7
      settings: SourceProductName=HDL Coder  SourceProductBaseCode=HD
  Minus : Sum  Inputs=3
  encoded_msg : Outport
  wires:
  basic_cycle/1 -> Bit Shift1/1
  Minus/1 -> encoded_msg/1
  tx_counter/1 -> Bit Shift/1
  Bit Shift1/1 -> Minus/1
  Bit Shift/1 -> Minus/2
  verif_value/1 -> Minus/3

== system HANcoder_E407_TTA_Controller_v4_7/HANcoder STM32 Target - E407-STM32 algorithm/TTA CAN System/TTA System/Matrix Cycle Manager/Vehicle Emulator Matrix Cycle/vehicle emulator basic cycle 1/COMM Task - Sync bc 1/Transmission subtasks/Check msg transmission CAN1/TX buffer update CAN1/Msg_Data_Encoder ==
  basic_cycle : Inport
  tx_counter : Inport  Port=2
  board_number : Inport  Port=3
  Bit Shift : hdlsllib/Logic and Bit Operations/Bit Shift  mode=Shift Left Logical  N=4
      settings: SourceProductName=HDL Coder  SourceProductBaseCode=HD
  Bit Shift1 : hdlsllib/Logic and Bit Operations/Bit Shift  mode=Shift Left Logical  N=7
      settings: SourceProductName=HDL Coder  SourceProductBaseCode=HD
  Minus : Sum  Inputs=3
  encoded_msg : Outport
  wires:
  basic_cycle/1 -> Bit Shift1/1
  Minus/1 -> encoded_msg/1
  tx_counter/1 -> Bit Shift/1
  Bit Shift1/1 -> Minus/1
  Bit Shift/1 -> Minus/2
  board_number/1 -> Minus/3

== system HANcoder_E407_TTA_Controller_v4_7/HANcoder STM32 Target - E407-STM32 algorithm/TTA CAN System/TTA System/Matrix Cycle Manager/Vehicle Emulator Matrix Cycle/vehicle emulator basic cycle 1/COMM Task - Sync bc 1/Transmission subtasks/Check msg transmission CAN2/TX buffer update CAN2/Msg_Data_Encoder ==
  basic_cycle : Inport
  tx_counter : Inport  Port=2
  verif_value : Inport  Port=3
  Bit Shift : hdlsllib/Logic and Bit Operations/Bit Shift  mode=Shift Left Logical  N=4
      settings: SourceProductName=HDL Coder  SourceProductBaseCode=HD
  Bit Shift1 : hdlsllib/Logic and Bit Operations/Bit Shift  mode=Shift Left Logical  N=7
      settings: SourceProductName=HDL Coder  SourceProductBaseCode=HD
  Minus : Sum  Inputs=3
  encoded_msg : Outport
  wires:
  basic_cycle/1 -> Bit Shift1/1
  Minus/1 -> encoded_msg/1
  tx_counter/1 -> Bit Shift/1
  Bit Shift1/1 -> Minus/1
  Bit Shift/1 -> Minus/2
  verif_value/1 -> Minus/3

== matlab function HANcoder_E407_TTA_Controller_v4_7/HANcoder STM32 Target - E407-STM32 algorithm/TTA CAN System/TTA System/LT_Update Desync_Positive/MATLAB Function ==
  data: local_time input; result_time output; TM_data input; TM_type input; phase_init1 input; phase1 input; phase_init2 input; phase2 input
%%% time_until_next_COMP
% receives current local_time (ticks) and returns how many ticks are left
% before the next computation. It also requires the Time Marks (TM) array
% and the type of task COMM (0) or COMP (1). 
% The definition of COMM and COMP is done in the _startup file for the
% simulink model.
% It is important to distinguish from one another because COMM tasks
% generate a send message every phase_1 or phase_2 ticks. 

function result_time = time_until_next_COMP(local_time, TM_data, TM_type,...
                                            phase_init1, phase1,...
                                            phase_init2, phase2)
    i = 1;
    % search iteratively over the TM array until the time window for the
    % local time is found:
    while local_time > TM_data(i)
        i = i+1;
    end
    
    if TM_type(i-1) % COMP -> 1
        % Ticks until next activation
        result_time = TM_data(i) - local_time - 1;
        
    else            % COMM -> 0
        % Time since the COMM task was activated
        COMM_local = local_time - TM_data(i-1);        
        % Closest next phase1 multiple
        next_send_mult_CAN1 =...
            (floor((COMM_local-phase_init1)/phase1) + 1)*phase1 + phase_init1;
        % Closest next phase2 multiple
        next_send_mult_CAN2 = ...
            (floor((COMM_local-phase_init2)/phase2) + 1)*phase2 + phase_init2;
        % We get when the next send is going to happen
        next_send = min(next_send_mult_CAN1,...
                        next_send_mult_CAN2);
        % And finally, the ticks until next send
        % <!> We should not skip the update buffer Tx task either! That is
        % we put -2 at the end.
        result_time = next_send - COMM_local - 2;
    end
end

== stateflow chart HANcoder_E407_TTA_Controller_v4_7/HANcoder STM32 Target - E407-STM32 algorithm/TTA CAN System/TTA System/Chart ==
  state Send_Trigger
    if (Condition)
    send(Trigger_Signal)
    end
  (default) -> Send_Trigger
  data: Condition input
  events: Trigger_Signal output FUNCTION_CALL_EVENT

== stateflow chart HANcoder_E407_TTA_Controller_v4_7/HANcoder STM32 Target - E407-STM32 algorithm/TTA CAN System/TTA System/Chart1 ==
  state Send_Trigger
    if (Condition)
    send(Trigger_Signal)
    end
  (default) -> Send_Trigger
  data: Condition input
  events: Trigger_Signal output FUNCTION_CALL_EVENT

== stateflow chart HANcoder_E407_TTA_Controller_v4_7/HANcoder STM32 Target - E407-STM32 algorithm/TTA CAN System/TTA System/Chart2 ==
  state Send_Trigger
    if (Condition)
    send(Trigger_Signal)
    end
  (default) -> Send_Trigger
  data: Condition input
  events: Trigger_Signal output FUNCTION_CALL_EVENT

== stateflow chart HANcoder_E407_TTA_Controller_v4_7/HANcoder STM32 Target - E407-STM32 algorithm/TTA CAN System/TTA System/Chart3 ==
  state Send_Trigger
    if (Condition)
    send(Trigger_Signal)
    end
  (default) -> Send_Trigger
  data: Condition input
  events: Trigger_Signal output FUNCTION_CALL_EVENT

== stateflow chart HANcoder_E407_TTA_Controller_v4_7/HANcoder STM32 Target - E407-STM32 algorithm/TTA CAN System/TTA System/Chart4 ==
  state Send_Trigger
    if (Condition)
    send(Trigger_Signal)
    end
  (default) -> Send_Trigger
  data: Condition input
  events: Trigger_Signal output FUNCTION_CALL_EVENT

== stateflow chart HANcoder_E407_TTA_Controller_v4_7/HANcoder STM32 Target - E407-STM32 algorithm/TTA CAN System/Local Time generation/Chart ==
  state Send_Trigger
    if (Condition)
    send(Trigger_Signal)
    end
  (default) -> Send_Trigger
  data: Condition input
  events: Trigger_Signal output FUNCTION_CALL_EVENT
